simulink model "aufgabe5_d"  (R2023a)
settings: Solver=ode45  StartTime=0.0  StopTime=5e-6  RelTol=1e-3
settings Model: Creator=ahm2d  LastModifiedBy=ahm2d

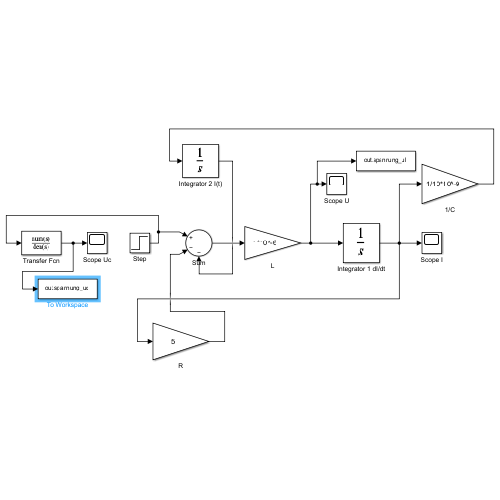
[thumbnail: Simulink's stored preview of the top-level diagram]
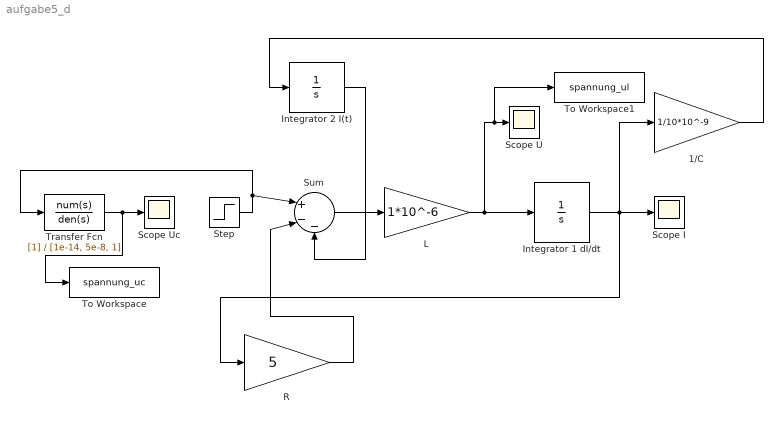
== system aufgabe5_d ==
  1/C : Gain  Gain=1/10*10^-9
  Integrator 1 dI/dt : Integrator
  Integrator 2 I(t) : Integrator
  L : Gain  Gain=1*10^-6
  R : Gain  Gain=5
  Scope I : Scope
  Scope U : Scope
  Scope Uc : Scope
  Step : Step  Time=0  SampleTime=0
  Sum : Sum  Inputs=|+--
  To Workspace : ToWorkspace  VariableName=spannung_uc  SampleTime=-1
  To Workspace1 : ToWorkspace  VariableName=spannung_ul  SampleTime=-1
  Transfer Fcn : TransferFcn  Denominator=[1e-14, 5e-8, 1]
  wires:
  Sum/1 -> L/1
  L/1 -> Integrator 1 dI/dt/1, To Workspace1/1, Scope U/1
  Integrator 1 dI/dt/1 -> R/1, Scope I/1, 1/C/1
  R/1 -> Sum/2
  1/C/1 -> Integrator 2 I(t)/1
  Step/1 -> Sum/1, Transfer Fcn/1
  Integrator 2 I(t)/1 -> Sum/3
  Transfer Fcn/1 -> To Workspace/1, Scope Uc/1
